simulink model "DC_PM_motor"  (R2019a)
settings: Solver=VariableStepAuto  StartTime=0.0  StopTime=10.0  RelTol=1e-3
values from neighbouring files (symbols this model uses):
  Jm = 0.05    [motorDC_matlab.m]
  Kd = (2 * ksi * wn + p - denH(2))/numH(3)    [motorDC_matlab.m]
  Ke = 0.4    [motorDC_matlab.m]
  Kf = 0.001    [motorDC_matlab.m]
  Ki = (p * wn^2)/numH(3)    [motorDC_matlab.m]
  Kp = (2 * p * ksi * wn + wn^2 - denH(3))/numH(3)    [motorDC_matlab.m]
  La = 10e-3    (= 0.01)    [motorDC_matlab.m]
  Ra = 0.5    [motorDC_matlab.m]
settings Model: Creator=User  LastModifiedBy=User
settings DebuggingCC: ArithmeticOperatorsInVariantConditions=warning

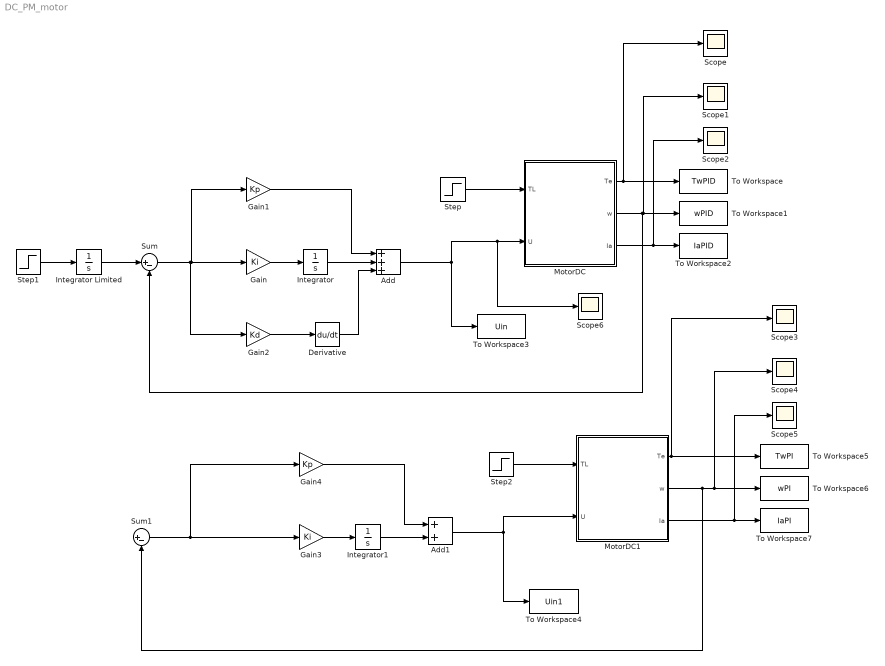
== system DC_PM_motor ==
  Add : Sum  Inputs=+++
  Add1 : Sum
  Derivative : Derivative
  Gain : Gain  Gain=Ki
  Gain1 : Gain  Gain=Kp
  Gain2 : Gain  Gain=Kd
  Gain3 : Gain  Gain=Ki
  Gain4 : Gain  Gain=Kp
  Integrator : Integrator
  Integrator Limited : Integrator  LimitOutput=on  UpperSaturationLimit=1  LowerSaturationLimit=0
  Integrator1 : Integrator
  MotorDC : Subsystem  Description=Motor DC
  MotorDC1 : Subsystem  Description=Motor DC
  Scope{,1..6} (7 alike) : Scope
  Step : Step  Time=5  SampleTime=0
  Step1 : Step  SampleTime=0
  Step2 : Step  SampleTime=0
  Sum : Sum  Inputs=|+-
  Sum1 : Sum  Inputs=|+-
  To Workspace : ToWorkspace  VariableName=TwPID  SaveFormat=Structure With Time  SampleTime=-1
  To Workspace1 : ToWorkspace  VariableName=wPID  SaveFormat=Structure With Time  SampleTime=-1
  To Workspace2 : ToWorkspace  VariableName=IaPID  SaveFormat=Structure With Time  SampleTime=-1
  To Workspace3 : ToWorkspace  VariableName=Uin  SaveFormat=Timeseries  SampleTime=-1
  To Workspace4 : ToWorkspace  VariableName=Uin1  SaveFormat=Timeseries  SampleTime=-1
  To Workspace5 : ToWorkspace  VariableName=TwPI  SaveFormat=Structure With Time  SampleTime=-1
  To Workspace6 : ToWorkspace  VariableName=wPI  SaveFormat=Structure With Time  SampleTime=-1
  To Workspace7 : ToWorkspace  VariableName=IaPI  SaveFormat=Structure With Time  SampleTime=-1
  wires:
  Step/1 -> MotorDC/1(TL)
  MotorDC/1(Te) -> Scope/1, To Workspace/1
  MotorDC/3(Ia) -> Scope2/1, To Workspace2/1
  Sum/1 -> Gain2/1, Gain1/1, Gain/1
  Gain/1 -> Integrator/1
  Integrator/1 -> Add/2
  Gain1/1 -> Add/1
  Add/1 -> To Workspace3/1, Scope6/1, MotorDC/2(U)
  MotorDC/2(w) -> Sum/2, Scope1/1, To Workspace1/1
  Add1/1 -> To Workspace4/1, MotorDC1/2(U)
  Gain3/1 -> Integrator1/1
  Integrator1/1 -> Add1/2
  Gain4/1 -> Add1/1
  Step2/1 -> MotorDC1/1(TL)
  Sum1/1 -> Gain4/1, Gain3/1
  MotorDC1/3(Ia) -> Scope5/1, To Workspace7/1
  MotorDC1/2(w) -> Sum1/2, Scope4/1, To Workspace6/1
  MotorDC1/1(Te) -> Scope3/1, To Workspace5/1
  Gain2/1 -> Derivative/1
  Derivative/1 -> Add/3
  Step1/1 -> Integrator Limited/1
  Integrator Limited/1 -> Sum/1

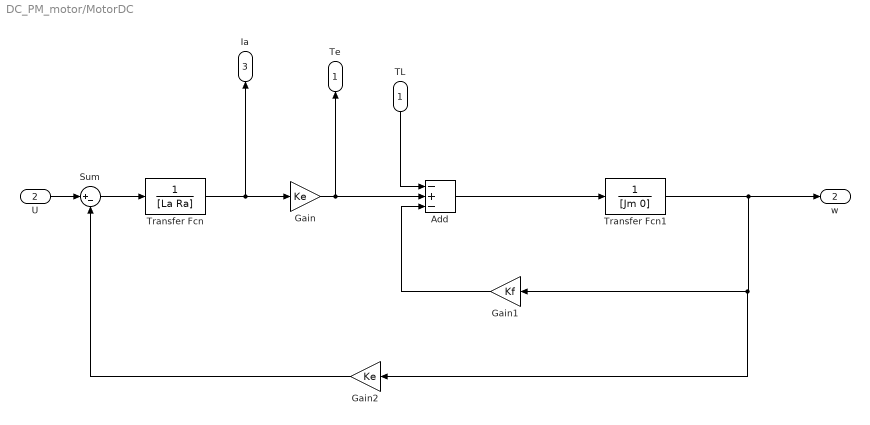
== system DC_PM_motor/MotorDC ==
  TL : Inport
  U : Inport  Port=2
  Add : Sum  Inputs=-+-
  Gain : Gain  Gain=Ke
  Gain1 : Gain  Gain=Kf
  Gain2 : Gain  Gain=Ke
  Sum : Sum  Inputs=|+-
  Transfer Fcn : TransferFcn  Denominator=[La Ra]
  Transfer Fcn1 : TransferFcn  Denominator=[Jm 0]
  Te : Outport
  w : Outport  Port=2
  Ia : Outport  Port=3
  wires:
  Sum/1 -> Transfer Fcn/1
  Transfer Fcn/1 -> Ia/1, Gain/1
  U/1 -> Sum/1
  Gain2/1 -> Sum/2
  Gain/1 -> Te/1, Add/2
  Gain1/1 -> Add/3
  TL/1 -> Add/1
  Add/1 -> Transfer Fcn1/1
  Transfer Fcn1/1 -> Gain2/1, Gain1/1, w/1

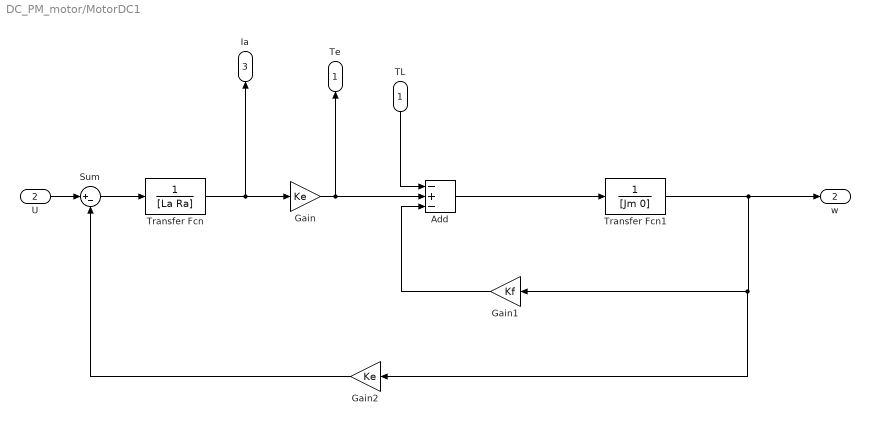
== system DC_PM_motor/MotorDC1 ==
  TL : Inport
  U : Inport  Port=2
  Add : Sum  Inputs=-+-
  Gain : Gain  Gain=Ke
  Gain1 : Gain  Gain=Kf
  Gain2 : Gain  Gain=Ke
  Sum : Sum  Inputs=|+-
  Transfer Fcn : TransferFcn  Denominator=[La Ra]
  Transfer Fcn1 : TransferFcn  Denominator=[Jm 0]
  Te : Outport
  w : Outport  Port=2
  Ia : Outport  Port=3
  wires:
  Sum/1 -> Transfer Fcn/1
  Transfer Fcn/1 -> Ia/1, Gain/1
  U/1 -> Sum/1
  Gain2/1 -> Sum/2
  Gain/1 -> Te/1, Add/2
  Gain1/1 -> Add/3
  TL/1 -> Add/1
  Add/1 -> Transfer Fcn1/1
  Transfer Fcn1/1 -> Gain2/1, Gain1/1, w/1
